simulink model "rtwdemo_autosar_PIM"  (Simulink 7.6)
settings: Solver=FixedStepDiscrete  StartTime=0.0  StopTime=10.0  FixedStep=0.01  RelTol=1e-3
PreLoadFcn:
  | rtwdemo_autosar_init_PIM
libraries: simulink x2, rtwlib x2
settings Model: Creator=The MathWorks Inc.
settings OptimizationCC: InlineParams=on  ZeroExternalMemoryAtStartup=off  ZeroInternalMemoryAtStartup=off  OptimizeModelRefInitCode=on  LifeSpan=1
settings DebuggingCC: InheritedTsInSrcMsg=none  StrictBusMsg=Warning
settings RTWCC: SystemTargetFile=autosar.tlc  GenCodeOnly=on  TemplateMakefile=ert_default_tmf  Description=Using Data Stores to Access Per-Instance Memory  GenerateReport=on  ProcessScript=autosar_make_rtw_hook  LaunchReport=on  GenerateCodeInfo=on
settings CodeAppCC: IgnoreCustomStorageClasses=off  SimulinkBlockComments=off
settings STFCustomTargetCC: ParMdlRefBuildCompliant=on  CompOptLevelCompliant=on  IncludeMdlTerminateFcn=off  CombineOutputUpdateFcns=on  SuppressErrorStatus=on  ERTFirstTimeCompliant=on  ERTCustomFileBanners=on  SupportNonFinite=off  SupportComplex=off  SupportContinuousTime=off  SupportNonInlinedSFcns=off  AutosarCompliant=on  SystemTargetFile=autosar.tlc
settings ERTTargetCC: MultiwordLength=2048  IncludeMdlTerminateFcn=off  SuppressErrorStatus=on  SupportNonFinite=off  SupportComplex=off  ModelStepFunctionPrototypeControlCompliant=off  CPPClassGenCompliant=off  AutosarCompliant=on  ExtModeMexFile=noextcomm  InlinedParameterPlacement=NonHierarchical  ERTCustomFileTemplate=example_file_process.tlc  ConvertIfToSwitch=off
settings CustomProperty: DataType=RTWOptions_EnumType__toolbox_rtw_targets_AUTOSAR_AUTOSAR_autosar_1_1AutosarSchemaVersion  Value=3.1
settings EnumStrPairs: String=2.0

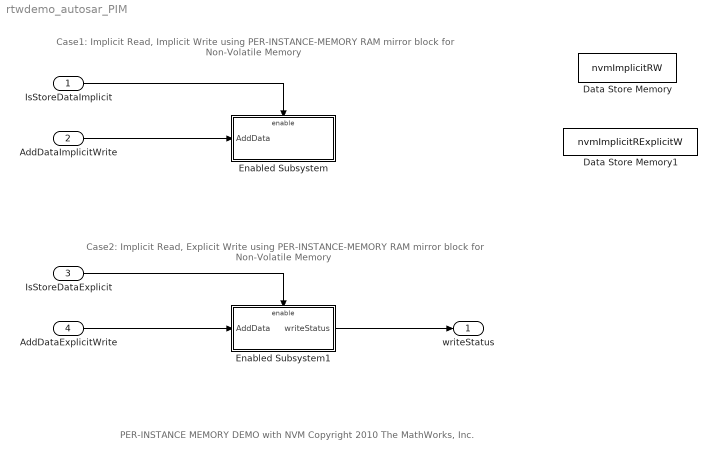
== system rtwdemo_autosar_PIM ==
  note: PER-INSTANCE MEMORY DEMO with NVM
      | Copyright 2010 The MathWorks, Inc.
  note: Case1: Implicit Read, Implicit Write
      | using PER-INSTANCE-MEMORY RAM mirror block for Non-Volatile Memory
  note: Case2: Implicit Read, Explicit Write
      | using PER-INSTANCE-MEMORY RAM mirror block for Non-Volatile Memory
  IsStoreDataImplicit : Inport  OutDataTypeStr=boolean
  AddDataImplicitWrite : Inport  Port=2
  IsStoreDataExplicit : Inport  Port=3  OutDataTypeStr=boolean
  AddDataExplicitWrite : Inport  Port=4
  Data Store Memory : DataStoreMemory  DataStoreName=nvmImplicitRW  ReadBeforeWriteMsg=warning  WriteAfterWriteMsg=warning  WriteAfterReadMsg=warning  StateMustResolveToSignalObject=on
  Data Store Memory1 : DataStoreMemory  DataStoreName=nvmImplicitRExplicitW  ReadBeforeWriteMsg=warning  WriteAfterWriteMsg=warning  WriteAfterReadMsg=warning  StateMustResolveToSignalObject=on
  Enabled Subsystem : Subsystem  TreatAsAtomicUnit=on
  Enabled Subsystem1 : Subsystem  TreatAsAtomicUnit=on
  writeStatus : Outport
  wires:
  IsStoreDataImplicit/1 -> Enabled Subsystem/Enable
  AddDataImplicitWrite/1 -> Enabled Subsystem/1(AddData)
  IsStoreDataExplicit/1 -> Enabled Subsystem1/Enable
  AddDataExplicitWrite/1 -> Enabled Subsystem1/1(AddData)
  Enabled Subsystem1/1(writeStatus) -> writeStatus/1

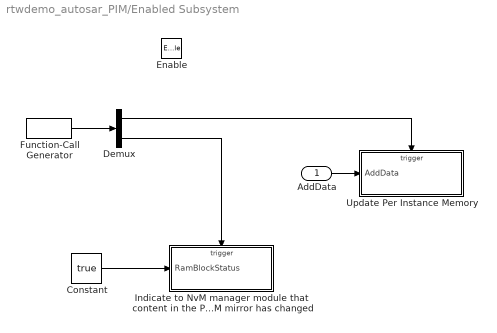
== system rtwdemo_autosar_PIM/Enabled Subsystem ==
  AddData : Inport
  Enable : EnablePort
  Constant : Constant  Value=true
  Demux : Demux  Outputs=2
  Function-Call Generator : simulink/Ports & Subsystems/Function-Call Generator  sample_time=-1  numberOfIterations=1
  Indicate to NvM manager module that  content in the PER-INSTANCE RAM mirror has changed : Subsystem  TreatAsAtomicUnit=on
  Update Per Instance Memory : Subsystem  TreatAsAtomicUnit=on
  wires:
  Function-Call Generator/1 -> Demux/1
  Demux/1 -> Update Per Instance Memory/Trigger
  Demux/2 -> Indicate to NvM manager module that  content in the PER-INSTANCE RAM mirror has changed/Trigger
  Constant/1 -> Indicate to NvM manager module that  content in the PER-INSTANCE RAM mirror has changed/1(RamBlockStatus)
  AddData/1 -> Update Per Instance Memory/1(AddData)

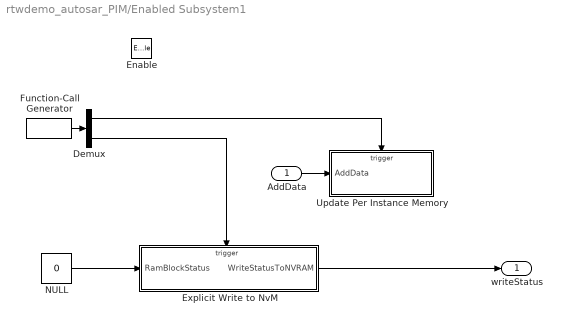
== system rtwdemo_autosar_PIM/Enabled Subsystem1 ==
  AddData : Inport
  Enable : EnablePort
  Demux : Demux  Outputs=2
  Explicit Write to NvM : Subsystem  TreatAsAtomicUnit=on
  Function-Call Generator : simulink/Ports & Subsystems/Function-Call Generator  sample_time=-1  numberOfIterations=1
  NULL : Constant  Value=0  OutDataTypeStr=uint8
  Update Per Instance Memory : Subsystem  TreatAsAtomicUnit=on
  writeStatus : Outport
  wires:
  AddData/1 -> Update Per Instance Memory/1(AddData)
  NULL/1 -> Explicit Write to NvM/1(RamBlockStatus)
  Demux/2 -> Explicit Write to NvM/Trigger
  Demux/1 -> Update Per Instance Memory/Trigger
  Function-Call Generator/1 -> Demux/1
  Explicit Write to NvM/1(WriteStatusToNVRAM) -> writeStatus/1

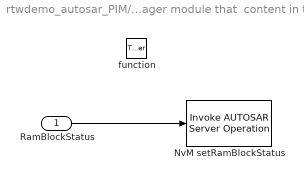
== system rtwdemo_autosar_PIM/Enabled Subsystem/Indicate to NvM manager module that  content in the PER-INSTANCE RAM mirror has changed ==
  RamBlockStatus : Inport
  function : TriggerPort  TriggerType=function-call
  NvM setRamBlockStatus : rtwlib/AUTOSAR/Invoke AUTOSAR Server Operation  portName=NvmService  operationPrototype=SetRamBlockStatus(IN boolean RamBlockStatus)  interfacePath=/AUTOSAR/Services/NvM  serverType=Basic software  showErrorStatus=off  SAMPLETIME=-1  showARPortLabels=on
  wires:
  RamBlockStatus/1 -> NvM setRamBlockStatus/1

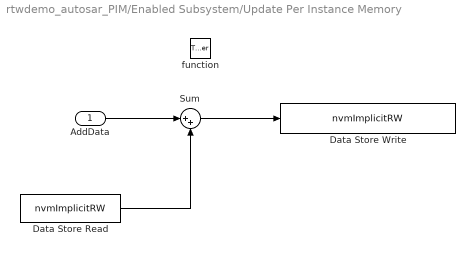
== system rtwdemo_autosar_PIM/Enabled Subsystem/Update Per Instance Memory ==
  AddData : Inport
  function : TriggerPort  TriggerType=function-call
  Data Store Read : DataStoreRead  DataStoreName=nvmImplicitRW
  Data Store Write : DataStoreWrite  DataStoreName=nvmImplicitRW
  Sum : Sum  Inputs=|++
  wires:
  AddData/1 -> Sum/1
  Data Store Read/1 -> Sum/2
  Sum/1 -> Data Store Write/1

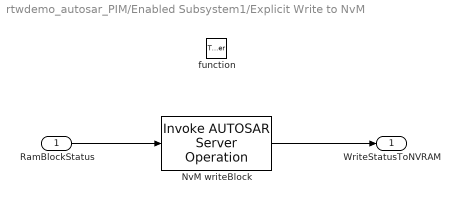
== system rtwdemo_autosar_PIM/Enabled Subsystem1/Explicit Write to NvM ==
  RamBlockStatus : Inport
  function : TriggerPort  TriggerType=function-call
  NvM writeBlock : rtwlib/AUTOSAR/Invoke AUTOSAR Server Operation  portName=NvmService  operationPrototype=WriteBlock(IN uint8 DstPtr)  interfacePath=/AUTOSAR/Services/NvM  serverType=Basic software  showErrorStatus=on  SAMPLETIME=-1  showARPortLabels=on
  WriteStatusToNVRAM : Outport
  wires:
  RamBlockStatus/1 -> NvM writeBlock/1
  NvM writeBlock/1 -> WriteStatusToNVRAM/1

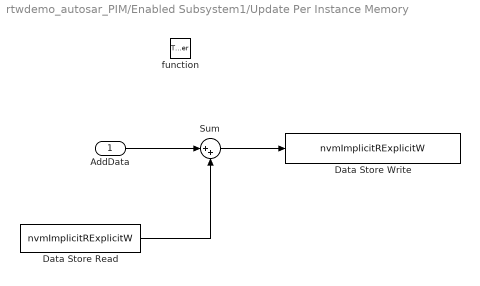
== system rtwdemo_autosar_PIM/Enabled Subsystem1/Update Per Instance Memory ==
  AddData : Inport
  function : TriggerPort  TriggerType=function-call
  Data Store Read : DataStoreRead  DataStoreName=nvmImplicitRExplicitW
  Data Store Write : DataStoreWrite  DataStoreName=nvmImplicitRExplicitW
  Sum : Sum  Inputs=|++
  wires:
  Sum/1 -> Data Store Write/1
  Data Store Read/1 -> Sum/2
  AddData/1 -> Sum/1
